simulink library "thrustlib"  (R2021b)
settings: Solver=VariableStepAuto  StartTime=0.0  StopTime=10.0  RelTol=1e-3
libraries: atmModelLib x1
settings Model: Creator=Triton  LastModifiedBy=Triton

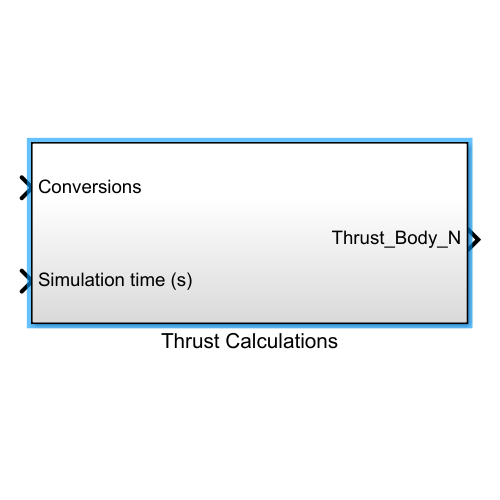
[thumbnail: Simulink's stored preview of the top-level diagram]
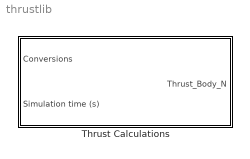
== system thrustlib ==
  Thrust Calculations : Subsystem

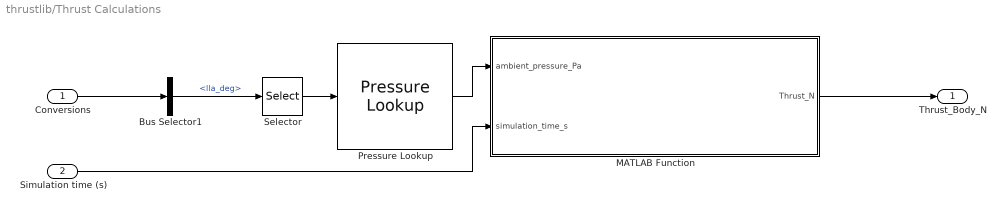
== system thrustlib/Thrust Calculations ==
  Conversions : Inport  OutDataTypeStr=Bus: Conversions_BusType
  Simulation time (s) : Inport  Port=2
  Bus Selector1 : BusSelector  OutputSignals=lla_deg
  MATLAB Function : MATLAB Function  TreatAsAtomicUnit=on
  Pressure Lookup : atmModelLib/Pressure Lookup  SystemSampleTime=-1  VariantActivationTime=update diagram  Latency=0  AutoFrameSizeCalculation=off
  Selector : Selector  InputPortWidth=3  IndexOptions=Index vector (dialog)  Indices=[3]  OutputSizes=1
  Thrust_Body_N : Outport
  wires:
  MATLAB Function/1(Thrust_N) -> Thrust_Body_N/1
  Selector/1 -> Pressure Lookup/1
  Pressure Lookup/1 -> MATLAB Function/1(ambient_pressure_Pa)
  Bus Selector1/1 -> Selector/1  "<lla_deg>"
  Conversions/1 -> Bus Selector1/1
  Simulation time (s)/1 -> MATLAB Function/2(simulation_time_s)

== matlab function thrustlib/Thrust Calculations/MATLAB Function ==
  data: Thrust_N output; ambient_pressure_Pa input; simulation_time_s input; Prop parameter
function Thrust_N = thrustVsPressure_wrapper(ambient_pressure_Pa, simulation_time_s, Prop)

if simulation_time_s < Prop.burn_time_s
    Thrust_N = thrustVsPressure(ambient_pressure_Pa, Prop);

else
    Thrust_N = [0;0;0];

end

end
